simulink model "narx"  (R2019a)
settings: Solver=VariableStepAuto  StartTime=0.0  StopTime=10.0  RelTol=1e-3
libraries: neural x208
(part 3 of 5)

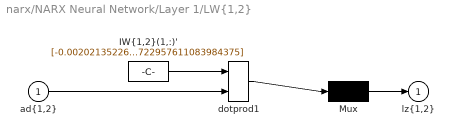
== system narx/NARX Neural Network/Layer 1/LW{1,2} ==
  "ad{1,2}" : Inport  PortDimensions=1600  SampleTime=0.1
      mask Display: e = 0.06;c1 = [120 230 180]/255;c2 = ([120 230 180]+0)/(256+128);c3 = ([120 230 180]+128)/(256+128);patch([0 1 1 0],[0 0 1 1],c1);patch([0 1 1 1-e 1-e 0+e],[0 0 1 1-e 0+e 0+e],c2);patch([0 0 1 1-e 0+e 0+e],[0 1 1 1-e 1-e 0+e],c3);plot([0 1 1 0 0],[0 0 1 1 0]);
  "IW{1,2}(1,:)'" : Constant  Value=[-0.0020213522679333024122116935217263744561932981014251708984375;0.02908660269959605082501497008706792257726192474365234375;0.0203283077947521116646267813621307141147553920745849609375;0.034636502273865492351756500966075691394507884979248046875;-0.0249326722769809654145500843469562823884189128875732421875;-0.023637576179618445537666815425836830399930477142333984375;0.0257148981615997369865045385495250229723751544952392578125;-0.03494418845822715169457950423748116008937358856201171875;0.038976946679742240087218618782571866177022457122802734375;-0.0366493212327144435302983538349508307874202728271484375;0.05259371834956085012269255685168900527060031890869140625;0.026317659979539505255008435824493062682449817657470703125;-0.040682931427733319551531820934542338363826274871826171875;0.0411851923372944794810024404796422459185123443603515625;0.05013682382187133190765138124334043823182582855224609375;0.008281903664360511230224659584564506076276302337646484375;-0.010550877427775766370654508818915928713977336883544921875;-0.005678799284663312019194592039639246650040149688720703125;0.0239411087387854902563955050709409988485276699066162109375;-0.0263563150685965676134348001369289704598486423492431640625;-0.0527230312316196714217397811808041296899318695068359375;0.051990100755978270463675272594628040678799152374267578125;0.0574799657220224913256600984823307953774929046630859375;0.03280195189588208659614565476658754050731658935546875;0.05670918413784682698963734992503304965794086456298828125;-0.0004455472041838672643716823262849402453866787254810333251953125;-0.041396459802379943770933579116899636574089527130126953125;-0.0030861347835023779200003257727757954853586852550506591796875;0.0286002860792995659833248822678797296248376369476318359375;0.020719316791316812198520125321010709740221500396728515625;0.043563977830384181810785548805142752826213836669921875;0.0303837531526354696909120178816010593436658382415771484375;0.01431694238504238776699128976588326622731983661651611328125;-0.0246737038150585154261396070296541438437998294830322265625;-0.0176625952251185103225594730247394181787967681884765625;0.039207076755730548012213176889417809434235095977783203125;-0.01202421439944922031128893280538250110112130641937255859375;-0.04682168642691812709966114880444365553557872772216796875;0.042607827002278324257655839346625725738704204559326171875;-0.0063881601688777593650581110296116094104945659637451171875;-0.0363741882096945967628442986097070388495922088623046875;-0.05548290330253495550305586903050425462424755096435546875;0.01833960045337990063529787221341393887996673583984375;-0.01386883816196017582544897095431224443018436431884765625;-0.0131389075789638161417816064613361959345638751983642578125;-0.005708389266597947188375261617920841672457754611968994140625;0.00280834037697736717265062367232530959881842136383056640625;-0.0217926744024648753883521834495695657096803188323974609375;-0.0014968924708328805971147001940835252753458917140960693359375;-0.055260839134774884795486826760679832659661769866943359375;-0.036447704942097543245882462770168785937130451202392578125;-0.021400544926688878921705594393642968498170375823974609375;0.02881363541160054941858703614343539811670780181884765625;0.01018477709372735649784313949339775717817246913909912109375;0.023887115740555138476697294436235097236931324005126953125;0.035669759772656239871224670423544012010097503662109375;0.041059051204006428992254740251155453734099864959716796875;-0.0425651552532213817148232237741467542946338653564453125;0.0188824841919854324867600325887906365096569061279296875;0.0297802208245369869066276891089728451333940029144287109375;0.0239920743035566715051221109433754463680088520050048828125;0.01294380700239725588696071412186938687227666378021240234375;-0.051614061388518588102680695328672300092875957489013671875;-0.03374689181365257695244253000055323354899883270263671875;-0.0183113842726967644691793424271963885985314846038818359375;0.0172390584396038375192272695812789606861770153045654296875 ...(+92896 chars)]
      mask Display: e = 0.06;c1 = [120 150 230]/255;c2 = ([120 150 230]+0)/383;c3 = ([120 150 230]+128)/383;patch([0 1 1 0],[0 0 1 1],c1);patch([0 1 1 1-e 1-e 0+e],[0 0 1 1-e 0+e 0+e],c2);patch([0 0 1 1-e 0+e 0+e],[0 1 1 1-e 1-e 0+e],c3);plot([0 1 1 0 0],[0 0 1 1 0]);disp('weights');
  Mux : Mux  Inputs=1
      mask Display: e = 0.06;c1 = [120 150 230]/255;c2 = ([120 150 230]+0)/383;c3 = ([120 150 230]+128)/383;patch([0 1 1 0],[0 0 1 1],c1);patch([0 1 1 1-e 1-e 0+e],[0 0 1 1-e 0+e 0+e],c2);patch([0 0 1 1-e 0+e 0+e],[0 1 1 1-e 1-e 0+e],c3);plot([0 1 1 0 0],[0 0 1 1 0]);disp('Mux');
  dotprod1 : neural/Weight Functions/dotprod
      settings: SourceProductName=MATLAB Runtime - Deep Learning Toolbox  SourceProductBaseCode=Missing
  "lz{1,2}" : Outport
      mask Display: e = 0.06;c1 = [120 230 180]/255;c2 = ([120 230 180]+0)/(256+128);c3 = ([120 230 180]+128)/(256+128);patch([0 1 1 0],[0 0 1 1],c1);patch([0 1 1 1-e 1-e 0+e],[0 0 1 1-e 0+e 0+e],c2);patch([0 0 1 1-e 0+e 0+e],[0 1 1 1-e 1-e 0+e],c3);plot([0 1 1 0 0],[0 0 1 1 0]);
  wires:
  "IW{1,2}(1,:)'"/1 -> dotprod1/1
  "ad{1,2}"/1 -> dotprod1/2
  dotprod1/1 -> Mux/1
  Mux/1 -> "lz{1,2}"/1
